simulink model "path_executor_test"  (Simulink 8.7)
settings: Solver=FixedStepAuto  StartTime=0.0  StopTime=35  FixedStep=0.01  RelTol=1e-3
libraries: simulink x1, tinbot x1
settings Model: Creator=eispin  LastModifiedBy=marlene
settings DataIOCC: LimitDataPoints=off  SaveFormat=Dataset
settings DebuggingCC: UnderspecifiedInitializationDetection=Simplified  MergeDetectMultiDrivingBlocksExec=error
settings HardwareCC: ProdBitPerPointer=64  ProdLargestAtomicFloat=Float  ProdIntDivRoundTo=Zero  ProdEndianess=LittleEndian  ProdWordSize=64  ProdHWDeviceType=Intel->x86-64 (Windows64)
settings ModelReferenceCC: PropagateSignalLabelsOutOfModel=on
settings ConfigComp: CovModelRefEnable=off

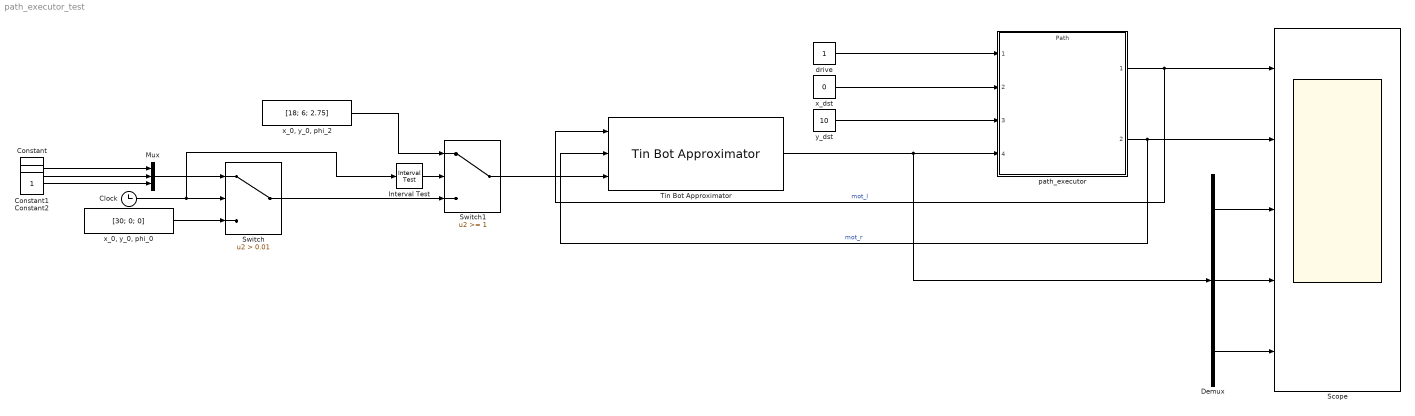
== system path_executor_test ==
  Clock : Clock
  Constant : Constant  Value=-1
  Constant1 : Constant
  Constant2 : Constant
  Demux : Demux  Outputs=3
  Interval Test : simulink/Logic and Bit Operations/Interval Test  IntervalClosedRight=on  uplimit=15  IntervalClosedLeft=on  lowlimit=14.8  OutDataTypeStr=boolean
  Mux : Mux  Inputs=3
  Scope : Scope  NumInputPorts=5
  Switch : Switch  Criteria=u2 > Threshold  Threshold=0.01
  Switch1 : Switch  Threshold=1
  Tin Bot Approximator : tinbot/Tin Bot Approximator  SystemSampleTime=-1
  drive : Constant
  path_executor : ModelReference  ModelNameDialog=Path.slx  SimulationMode=Normal  ModelReferenceVersion=1.40
  "x_0, y_0, phi_0" : Constant  Value=[30; 0; 0]
  "x_0, y_0, phi_2" : Constant  Value=[18; 6; 2.75]
  x_dst : Constant  Value=0
  y_dst : Constant  Value=10
  wires:
  drive/1 -> path_executor/1
  x_dst/1 -> path_executor/2
  y_dst/1 -> path_executor/3
  Tin Bot Approximator/1 -> Demux/1, path_executor/4
  path_executor/1 -> Tin Bot Approximator/1, Scope/1  "mot_l"
  path_executor/2 -> Tin Bot Approximator/2, Scope/2  "mot_r"
  "x_0, y_0, phi_0"/1 -> Switch/3
  Clock/1 -> Interval Test/1, Switch/2
  Mux/1 -> Switch/1
  Constant/1 -> Mux/1
  Constant1/1 -> Mux/2
  Constant2/1 -> Mux/3
  Switch/1 -> Switch1/3
  Interval Test/1 -> Switch1/2
  "x_0, y_0, phi_2"/1 -> Switch1/1
  Switch1/1 -> Tin Bot Approximator/3
  Demux/2 -> Scope/4
  Demux/1 -> Scope/3
  Demux/3 -> Scope/5
